simulink model "DiffBotControl"  (R2021a)
settings: Solver=ode45  StartTime=0.0  StopTime=20  RelTol=1e-3  EnableMultiTasking=on
values from neighbouring files (symbols this model uses):
  Tstep = 0.01    [PathFollowingMain.m]
  x0 = -1    [PathFollowingMain.m]
libraries: simulink x1
settings Model: Creator=Gu  LastModifiedBy=duong
settings SolverCC: AlgebraicLoopSolver=TrustRegion
settings DataIOCC: LimitDataPoints=on  SaveFormat=Array  SignalLoggingSaveFormat=ModelDataLogs  ReturnWorkspaceOutputs=off
settings OptimizationCC: ExpressionDepthLimit=2147483647  LifeSpan=inf
settings DebuggingCC: UnderspecifiedInitializationDetection=Classic  MergeDetectMultiDrivingBlocksExec=none  FcnCallInpInsideContextMsg=warning  StateNameClashWarn=warning  SFUnexpectedBacktrackingDiag=warning  SFNoUnconditionalDefaultTransitionDiag=warning  SFMachineParentedDataDiag=warning  ArithmeticOperatorsInVariantConditions=warning
settings HardwareCC: ProdBitPerPointer=32  ProdBitPerSizeT=32  ProdBitPerPtrDiffT=32  ProdLargestAtomicFloat=None  ProdIntDivRoundTo=Undefined  ProdEndianess=Unspecified  ProdWordSize=32  ProdHWDeviceType=32-bit Generic
settings ModelReferenceCC: PropagateSignalLabelsOutOfModel=off
settings SFSimCC: SimUseLocalCustomCode=off  SimParseCustomCode=off  CustomCodeUndefinedFunction=UseInterfaceOnly
settings RTWCC: RTWUseLocalCustomCode=off
settings CodeAppCC: StateflowObjectComments=on
settings GRTTargetCC: TargetLangStandard=C89/C90 (ANSI)  CombineOutputUpdateFcns=off  GRTInterface=on
settings ConfigComp: CovMetricSettings=dw  CovSaveCumulativeToWorkspaceVar=on  CovSaveSingleToWorkspaceVar=on  CovExternalEMLEnable=off  CovSFcnEnable=off

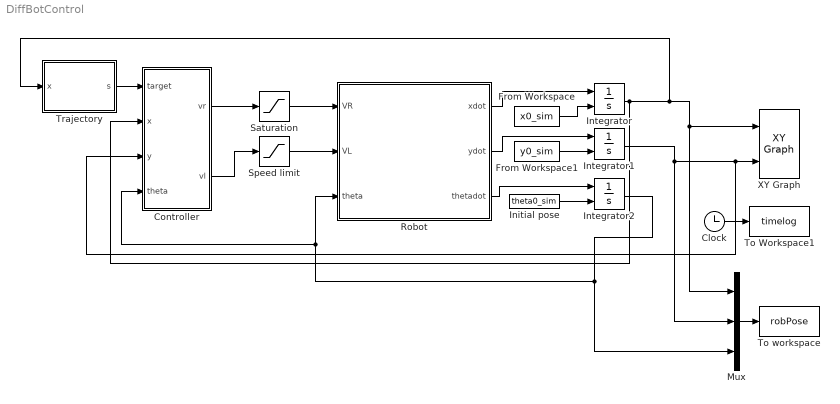
== system DiffBotControl ==
  Clock : Clock
  Controller : MATLAB Function  TreatAsAtomicUnit=on
  From Workspace : FromWorkspace  VariableName=x0_sim  OutputAfterFinalValue=Holding final value
  From Workspace1 : FromWorkspace  VariableName=y0_sim  OutputAfterFinalValue=Holding final value
  Initial pose : FromWorkspace  VariableName=theta0_sim  OutputAfterFinalValue=Holding final value
  Integrator : Integrator  InitialConditionSource=external  InitialCondition=x0
  Integrator1 : Integrator  InitialConditionSource=external  InitialCondition=2
  Integrator2 : Integrator  InitialConditionSource=external  InitialCondition=pi/4
  Mux : Mux  Inputs=3
  Robot : MATLAB Function  TreatAsAtomicUnit=on
  Saturation : Saturate  UpperLimit=1  LowerLimit=-1
  Speed limit : Saturate  UpperLimit=1  LowerLimit=-1
  To Workspace1 : ToWorkspace  VariableName=timelog  SampleTime=-1
      settings: Save2DSignal=2-D array (concatenate along first dimension)
  To workspace : ToWorkspace  VariableName=robPose  SampleTime=Tstep
  Trajectory : MATLAB Function  TreatAsAtomicUnit=on
  XY Graph : simulink/Sinks/XY Graph  xmin=-10  xmax=10  ymin=-10  ymax=10  st=-1
  wires:
  Robot/1(xdot) -> Integrator/1
  Robot/2(ydot) -> Integrator1/1
  Robot/3(thetadot) -> Integrator2/1
  Integrator2/1 -> Controller/4(theta), Robot/3(theta), Mux/3
  Integrator/1 -> Controller/2(x), Trajectory/1(x), XY Graph/1, Mux/1
  Integrator1/1 -> Controller/3(y), XY Graph/2, Mux/2
  Clock/1 -> To Workspace1/1
  Mux/1 -> To workspace/1
  From Workspace/1 -> Integrator/2
  From Workspace1/1 -> Integrator1/2
  Initial pose/1 -> Integrator2/2
  Trajectory/1(s) -> Controller/1(target)
  Controller/1(vr) -> Saturation/1
  Saturation/1 -> Robot/1(VR)
  Controller/2(vl) -> Speed limit/1
  Speed limit/1 -> Robot/2(VL)

== matlab function DiffBotControl/Controller ==
  data: vr output; target input; vl output; x input; y input; theta input
function [vr,vl] = fcn(target,x,y,theta)

% Control parameters
gamma=3;
lamda=6;
h=1;

% Target movement parameters
k=0.01;
ep=0.1;

% Robot parameter: Distance between two wheels
d=0.5;

% Calculate polar variables
rho = sqrt((target(1)-x)^2+(target(2)-y)^2);
phi = atan2(target(2)-y,target(1)-x)-target(3);
alpha = phi+target(3)-theta;

% Calculate control laws
v = gamma*cos(alpha)*rho;
w = lamda*alpha + gamma*cos(alpha)*sin(alpha)/alpha*(alpha+h*phi);

% Calculate Vl and Vr from v and w
vl = (2*v-d*w)/2;
vr = (2*v+d*w)/2;
end

== matlab function DiffBotControl/Robot ==
  data: VR input; xdot output; VL input; theta input; ydot output; thetadot output
function [xdot, ydot, thetadot] = fcn(VR, VL,theta)

d=0.5; % axial space
xdot=(VR+VL)/2*cos(theta);
ydot=(VR+VL)/2*sin(theta);
thetadot=(VR-VL)/d;

== matlab function DiffBotControl/Trajectory ==
  data: x input; s output
% Simply moving the target by a distance L
function s = fcn(x)
    f=@(x) atan(x^2); % The trajectory function being tracked
    L = 0.1;
    s = zeros(1,3);
    s(1) = x + L; % update target x
    s(2) = f(s(1)^2); % calculate target y based on the function used
    x_diff = s(1)-0.001;
    s(3) = atan2(s(2)-f(x_diff^2),s(1)-x_diff); % The angle is chosen as tangent vector
end
